simulink subsystem "AnglesdEulerA"  (R2023a)
settings: Solver=VariableStepAuto  StartTime=0.0  StopTime=10.0  RelTol=1e-3
settings Model: Creator=user  LastModifiedBy=raphb

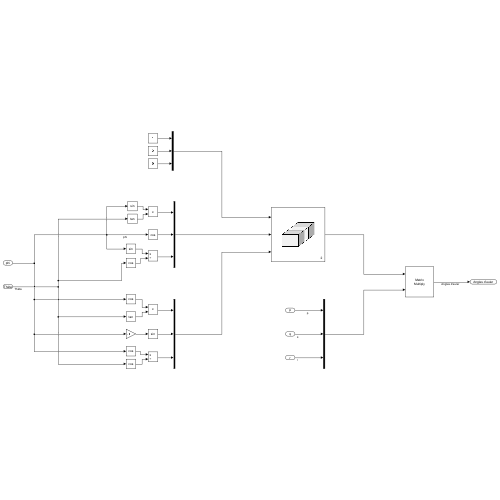
[thumbnail: Simulink's stored preview of the top-level diagram]
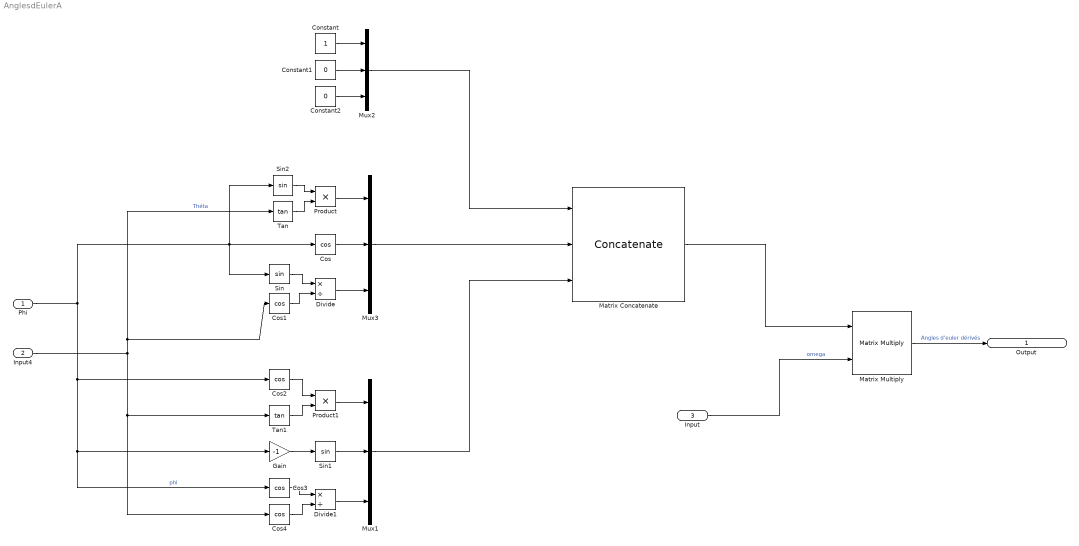
== system AnglesdEulerA ==
  Phi : Inport
  Input4 : Inport  Port=2
  Input : Inport  Port=3
  Constant : Constant
  Constant1 : Constant  Value=0
  Constant2 : Constant  Value=0
  Cos{,1..4} (5 alike) : Trigonometry  Operator=cos
  Divide : Product  Inputs=*/  RndMeth=Zero  SaturateOnIntegerOverflow=on
  Divide1 : Product  Inputs=*/
  Gain : Gain  Gain=-1
  Matrix Concatenate : Concatenate  NumInputs=3  Mode=Multidimensional array  ConcatenateDimension=2
  Matrix Multiply : Product  Multiplication=Matrix(*)
  Mux1 : Mux  Inputs=3
  Mux2 : Mux  Inputs=3
  Mux3 : Mux  Inputs=3
  Product : Product
  Product1 : Product
  Sin : Trigonometry
  Sin1 : Trigonometry
  Sin2 : Trigonometry
  Tan : Trigonometry  Operator=tan
  Tan1 : Trigonometry  Operator=tan
  Output : Outport
  wires:
  Constant/1 -> Mux2/1
  Constant1/1 -> Mux2/2
  Constant2/1 -> Mux2/3
  Phi/1 -> Cos3/1, Gain/1, Cos2/1, Sin2/1, Sin/1, Cos/1  "phi"
  Cos/1 -> Mux3/2
  Sin2/1 -> Product/1
  Input4/1 -> Tan/1, Cos1/1, Cos4/1, Tan1/1  "Théta"
  Tan/1 -> Product/2
  Product/1 -> Mux3/1
  Cos1/1 -> Divide/2
  Sin/1 -> Divide/1
  Divide/1 -> Mux3/3
  Tan1/1 -> Product1/2
  Cos2/1 -> Product1/1
  Product1/1 -> Mux1/1
  Gain/1 -> Sin1/1
  Sin1/1 -> Mux1/2
  Cos3/1 -> Divide1/1
  Cos4/1 -> Divide1/2
  Divide1/1 -> Mux1/3
  Mux2/1 -> Matrix Concatenate/1
  Mux3/1 -> Matrix Concatenate/2
  Mux1/1 -> Matrix Concatenate/3
  Matrix Concatenate/1 -> Matrix Multiply/1
  Matrix Multiply/1 -> Output/1  "Angles d’euler dérivés"
  Input/1 -> Matrix Multiply/2  "omega"
